simulink model "cm_sat_model"  (R2021b)
settings: Solver=ode23s  StartTime=0.0  StopTime=0.2  FixedStep=0.0001  MaxStep=1e-3  RelTol=5e-7  AbsTol=5e-7  EnableMultiTasking=on
values from neighbouring files (symbols this model uses):
  Rn = 10    [sim_cm_sat.m]
  VA = sqrt(2)*120    [sim_cm_sat.m]
  VAf = 0    [sim_cm_sat.m]
  VB = VA    [sim_cm_sat.m]
  VBf = (2*pi)/3    (= 2.09439510239)    [sim_cm_sat.m]
  VC = VB    [sim_cm_sat.m]
  VCf = (4*pi)/3    (= 4.18879020479)    [sim_cm_sat.m]
undefined symbols (not defined in the file or in its folder): Dpsi, PAR, psisat, wb, XINIT
settings Model: Creator=Alberto  LastModifiedBy=Usuario
settings SolverCC: AutoScaleAbsTol=off  MaxOrder=4  AlgebraicLoopSolver=TrustRegion
settings DataIOCC: LimitDataPoints=on  SaveFormat=Array  SignalLoggingSaveFormat=ModelDataLogs  ReturnWorkspaceOutputs=off  SignalLoggingName=sigsOut
settings OptimizationCC: ExpressionDepthLimit=2147483647  LifeSpan=inf
settings DebuggingCC: AlgebraicLoopMsg=none  SaveWithParameterizedLinksMsg=none  UnderspecifiedInitializationDetection=Classic  MergeDetectMultiDrivingBlocksExec=none  SignalResolutionControl=TryResolveAllWithWarning  MultiTaskDSMMsg=warning  MultiTaskCondExecSysMsg=none  FcnCallInpInsideContextMsg=warning  StateNameClashWarn=warning  SFUnexpectedBacktrackingDiag=warning  SFNoUnconditionalDefaultTransitionDiag=warning  SFExecutionAtInitializationDiag=none  SFMachineParentedDataDiag=warning  ArithmeticOperatorsInVariantConditions=warning
settings HardwareCC: ProdBitPerPointer=32  ProdBitPerSizeT=32  ProdBitPerPtrDiffT=32  ProdLargestAtomicFloat=None  ProdIntDivRoundTo=Undefined  ProdEndianess=Unspecified  ProdWordSize=32  ProdHWDeviceType=32-bit Generic  TargetUnknown=on
settings ModelReferenceCC: PropagateSignalLabelsOutOfModel=off
settings SFSimCC: SimUseLocalCustomCode=off  CustomCodeUndefinedFunction=UseInterfaceOnly
settings RTWCC: RTWUseLocalCustomCode=off
settings CodeAppCC: StateflowObjectComments=on
settings GRTTargetCC: TargetLangStandard=C89/C90 (ANSI)  CombineOutputUpdateFcns=off  GRTInterface=on
settings ConfigComp: CovMetricSettings=dw  CovSaveCumulativeToWorkspaceVar=on  CovSaveSingleToWorkspaceVar=on  CovExternalEMLEnable=off

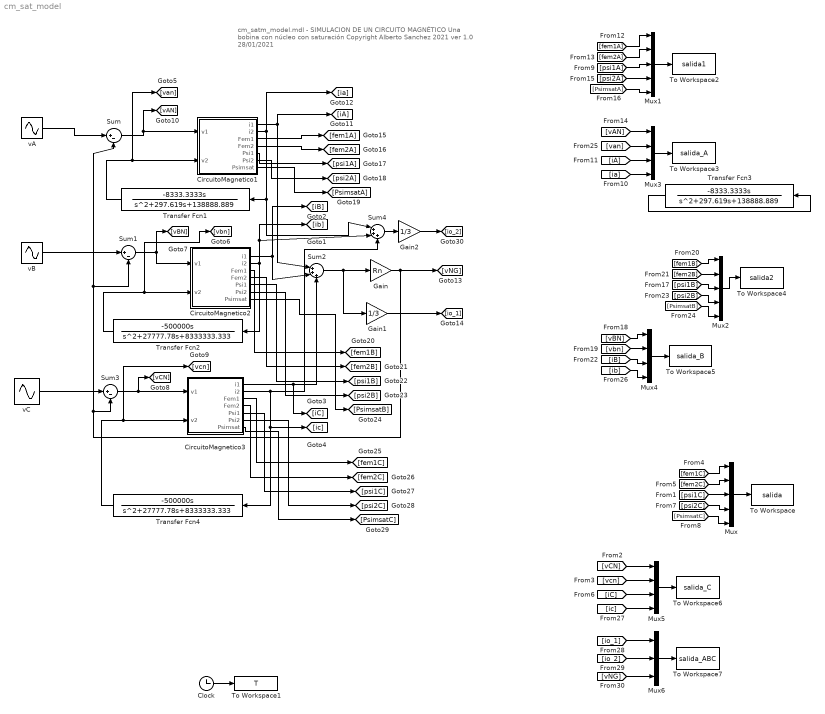
== system cm_sat_model ==
  note: cm_satm_model.mdl - SIMULACION DE UN CIRCUITO MAGNÉTICO
      | Una bobina con núcleo con saturación
      | Copyright Alberto Sanchez 2021
      | ver 1.0 28/01/2021
  CircuitoMagnetico1 : Subsystem
  CircuitoMagnetico2 : Subsystem
  CircuitoMagnetico3 : Subsystem
  Clock : Clock
  Gain : Gain  Gain=Rn
  Gain1 : Gain  Gain=1/3
  Gain2 : Gain  Gain=1/3
  Mux : Mux  Inputs=5
  Mux1 : Mux  Inputs=5
  Mux2 : Mux  Inputs=5
  Mux3 : Mux
  Mux4 : Mux
  Mux5 : Mux
  Mux6 : Mux  Inputs=3
  Sum : Sum  Inputs=|+-
  Sum1 : Sum  Inputs=|+-
  Sum2 : Sum  Inputs=|+++
  Sum3 : Sum  Inputs=|+-
  Sum4 : Sum  Inputs=|+++
  To Workspace : ToWorkspace  VariableName=salida  SampleTime=-1
  To Workspace1 : ToWorkspace  VariableName=T  SampleTime=-1
  To Workspace2 : ToWorkspace  VariableName=salida1  SampleTime=-1
  To Workspace3 : ToWorkspace  VariableName=salida_A  SampleTime=-1
  To Workspace4 : ToWorkspace  VariableName=salida2  SampleTime=-1
  To Workspace5 : ToWorkspace  VariableName=salida_B  SampleTime=-1
  To Workspace6 : ToWorkspace  VariableName=salida_C  SampleTime=-1
  To Workspace7 : ToWorkspace  VariableName=salida_ABC  SampleTime=-1
  Transfer Fcn1 : TransferFcn  Numerator=[-8333.3333 0]  Denominator=[1 297.619 138888.889]
  Transfer Fcn2 : TransferFcn  Numerator=[-500000 0]  Denominator=[1 27777.78 8333333.333]
  Transfer Fcn3 : TransferFcn  Numerator=[-8333.3333 0]  Denominator=[1 297.619 138888.889]
  Transfer Fcn4 : TransferFcn  Numerator=[-500000 0]  Denominator=[1 27777.78 8333333.333]
  vA : Sin  Amplitude=VA  Frequency=wb  Phase=VAf  SampleTime=0
  vB : Sin  Amplitude=VB  Frequency=wb  Phase=VBf  SampleTime=0
  vC : Sin  Amplitude=VC  Frequency=wb  Phase=VCf  SampleTime=0
  wires:
  Mux1/1 -> To Workspace2/1
  Mux2/1 -> To Workspace4/1
  Mux/1 -> To Workspace/1
  Clock/1 -> To Workspace1/1
  [fem1B] -> Mux2/1
  [fem2B] -> Mux2/2
  [psi1B] -> Mux2/3
  [psi2B] -> Mux2/4
  [PsimsatB] -> Mux2/5
  [fem1A] -> Mux1/1
  [fem2A] -> Mux1/2
  [psi1A] -> Mux1/3
  [psi2A] -> Mux1/4
  [PsimsatA] -> Mux1/5
  [fem1C] -> Mux/1
  [fem2C] -> Mux/2
  [psi1C] -> Mux/3
  [psi2C] -> Mux/4
  [PsimsatC] -> Mux/5
  [vAN] -> Mux3/1
  [van] -> Mux3/2
  [iA] -> Mux3/3
  [ia] -> Mux3/4
  Mux3/1 -> To Workspace3/1
  Mux4/1 -> To Workspace5/1
  [vbn] -> Mux4/2
  [vBN] -> Mux4/1
  [iB] -> Mux4/3
  [ib] -> Mux4/4
  Mux5/1 -> To Workspace6/1
  [vCN] -> Mux5/1
  [vcn] -> Mux5/2
  [iC] -> Mux5/3
  [ic] -> Mux5/4
  Mux6/1 -> To Workspace7/1
  Transfer Fcn3/1 -> Transfer Fcn3/1
  Sum/1 -> CircuitoMagnetico1/1(v1), [vAN]
  Transfer Fcn4/1 -> [vcn], CircuitoMagnetico3/2(v2)
  Transfer Fcn2/1 -> [vbn], CircuitoMagnetico2/2(v2)
  CircuitoMagnetico2/5(Psi1) -> [psi1B]
  vC/1 -> Sum3/1
  CircuitoMagnetico2/4(Fem2) -> [fem2B]
  CircuitoMagnetico2/1(i1) -> Sum2/2, [iB]
  Sum2/1 -> Gain1/1, Gain/1
  CircuitoMagnetico3/3(Fem1) -> [fem1C]
  CircuitoMagnetico3/4(Fem2) -> [fem2C]
  CircuitoMagnetico1/5(Psi1) -> [psi1A]
  CircuitoMagnetico1/2(i2) -> Transfer Fcn1/1, Sum4/1, [ia]
  CircuitoMagnetico3/6(Psi2) -> [psi2C]
  CircuitoMagnetico3/2(i2) -> Sum4/3, Transfer Fcn4/1, [ic]
  CircuitoMagnetico2/7(Psimsat) -> [PsimsatB]
  Sum3/1 -> [vCN], CircuitoMagnetico3/1(v1)
  Gain1/1 -> [io_1]
  CircuitoMagnetico2/3(Fem1) -> [fem1B]
  CircuitoMagnetico1/4(Fem2) -> [fem2A]
  CircuitoMagnetico1/6(Psi2) -> [psi2A]
  CircuitoMagnetico3/5(Psi1) -> [psi1C]
  Gain/1 -> [vNG], Sum1/2, Sum/2, Sum3/2
  CircuitoMagnetico3/7(Psimsat) -> [PsimsatC]
  CircuitoMagnetico2/2(i2) -> Transfer Fcn2/1, Sum4/2, [ib]
  CircuitoMagnetico1/1(i1) -> Sum2/1, [iA]
  CircuitoMagnetico1/7(Psimsat) -> [PsimsatA]
  vB/1 -> Sum1/1
  Sum1/1 -> CircuitoMagnetico2/1(v1), [vBN]
  CircuitoMagnetico2/6(Psi2) -> [psi2B]
  CircuitoMagnetico1/3(Fem1) -> [fem1A]
  CircuitoMagnetico3/1(i1) -> Sum2/3, [iC]
  vA/1 -> Sum/1
  Transfer Fcn1/1 -> [van], CircuitoMagnetico1/2(v2)
  Sum4/1 -> Gain2/1
  Gain2/1 -> [io_2]
  [io_2] -> Mux6/2
  [io_1] -> Mux6/1
  [vNG] -> Mux6/3

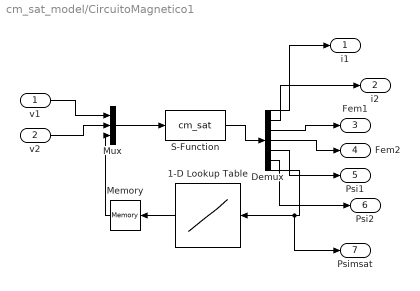
== system cm_sat_model/CircuitoMagnetico1 ==
  v1 : Inport
  v2 : Inport  Port=2
  1-D Lookup Table : Lookup_n-D  NumberOfTableDimensions=1  BreakpointsForDimension1=psisat  Table=Dpsi  RndMeth=Simplest  InputSameDT=on
  Demux : Demux  Outputs=7
      settings: DisplayOption=none
  Memory : Memory
  Mux : Mux  Inputs=3
  S-Function : S-Function  FunctionName=cm_sat  Parameters=XINIT,PAR  SFunctionDeploymentMode=off  EnableBusSupport=off
  i1 : Outport  VectorParamsAs1DForOutWhenUnconnected=off
  i2 : Outport  Port=2  VectorParamsAs1DForOutWhenUnconnected=off
  Fem1 : Outport  Port=3  VectorParamsAs1DForOutWhenUnconnected=off
  Fem2 : Outport  Port=4  VectorParamsAs1DForOutWhenUnconnected=off
  Psi1 : Outport  Port=5  VectorParamsAs1DForOutWhenUnconnected=off
  Psi2 : Outport  Port=6  VectorParamsAs1DForOutWhenUnconnected=off
  Psimsat : Outport  Port=7  VectorParamsAs1DForOutWhenUnconnected=off
  wires:
  v2/1 -> Mux/2
  Demux/4 -> Fem2/1
  Demux/2 -> i2/1
  Memory/1 -> Mux/3
  Demux/6 -> Psi2/1
  S-Function/1 -> Demux/1
  Demux/7 -> 1-D Lookup Table/1, Psimsat/1
  Demux/3 -> Fem1/1
  Demux/1 -> i1/1
  Demux/5 -> Psi1/1
  v1/1 -> Mux/1
  Mux/1 -> S-Function/1
  1-D Lookup Table/1 -> Memory/1

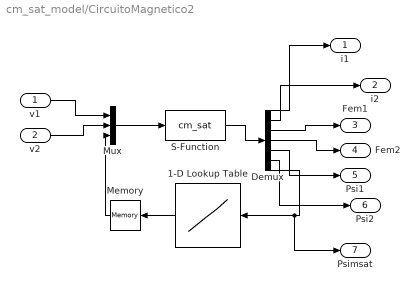
== system cm_sat_model/CircuitoMagnetico2 ==
  v1 : Inport
  v2 : Inport  Port=2
  1-D Lookup Table : Lookup_n-D  NumberOfTableDimensions=1  BreakpointsForDimension1=psisat  Table=Dpsi  RndMeth=Simplest  InputSameDT=on
  Demux : Demux  Outputs=7
      settings: DisplayOption=none
  Memory : Memory
  Mux : Mux  Inputs=3
  S-Function : S-Function  FunctionName=cm_sat  Parameters=XINIT,PAR  SFunctionDeploymentMode=off  EnableBusSupport=off
  i1 : Outport  VectorParamsAs1DForOutWhenUnconnected=off
  i2 : Outport  Port=2  VectorParamsAs1DForOutWhenUnconnected=off
  Fem1 : Outport  Port=3  VectorParamsAs1DForOutWhenUnconnected=off
  Fem2 : Outport  Port=4  VectorParamsAs1DForOutWhenUnconnected=off
  Psi1 : Outport  Port=5  VectorParamsAs1DForOutWhenUnconnected=off
  Psi2 : Outport  Port=6  VectorParamsAs1DForOutWhenUnconnected=off
  Psimsat : Outport  Port=7  VectorParamsAs1DForOutWhenUnconnected=off
  wires:
  v2/1 -> Mux/2
  Demux/4 -> Fem2/1
  Demux/2 -> i2/1
  Memory/1 -> Mux/3
  Demux/6 -> Psi2/1
  S-Function/1 -> Demux/1
  Demux/7 -> 1-D Lookup Table/1, Psimsat/1
  Demux/3 -> Fem1/1
  Demux/1 -> i1/1
  Demux/5 -> Psi1/1
  v1/1 -> Mux/1
  Mux/1 -> S-Function/1
  1-D Lookup Table/1 -> Memory/1

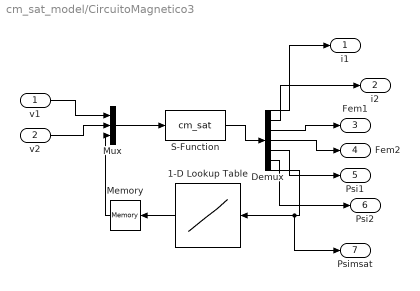
== system cm_sat_model/CircuitoMagnetico3 ==
  v1 : Inport
  v2 : Inport  Port=2
  1-D Lookup Table : Lookup_n-D  NumberOfTableDimensions=1  BreakpointsForDimension1=psisat  Table=Dpsi  RndMeth=Simplest  InputSameDT=on
  Demux : Demux  Outputs=7
      settings: DisplayOption=none
  Memory : Memory
  Mux : Mux  Inputs=3
  S-Function : S-Function  FunctionName=cm_sat  Parameters=XINIT,PAR  SFunctionDeploymentMode=off  EnableBusSupport=off
  i1 : Outport  VectorParamsAs1DForOutWhenUnconnected=off
  i2 : Outport  Port=2  VectorParamsAs1DForOutWhenUnconnected=off
  Fem1 : Outport  Port=3  VectorParamsAs1DForOutWhenUnconnected=off
  Fem2 : Outport  Port=4  VectorParamsAs1DForOutWhenUnconnected=off
  Psi1 : Outport  Port=5  VectorParamsAs1DForOutWhenUnconnected=off
  Psi2 : Outport  Port=6  VectorParamsAs1DForOutWhenUnconnected=off
  Psimsat : Outport  Port=7  VectorParamsAs1DForOutWhenUnconnected=off
  wires:
  v2/1 -> Mux/2
  Demux/4 -> Fem2/1
  Demux/2 -> i2/1
  Memory/1 -> Mux/3
  Demux/6 -> Psi2/1
  S-Function/1 -> Demux/1
  Demux/7 -> 1-D Lookup Table/1, Psimsat/1
  Demux/3 -> Fem1/1
  Demux/1 -> i1/1
  Demux/5 -> Psi1/1
  v1/1 -> Mux/1
  Mux/1 -> S-Function/1
  1-D Lookup Table/1 -> Memory/1
